simulink library "pixhawk_slib_rfly"  (R2022b)
settings: Solver=ode45  StartTime=0.0  StopTime=10.0  RelTol=1e-3
libraries: pixhawk_slib_uORB_RW x42, $bdroot x7
(part 3 of 3)

== matlab function pixhawk_slib_rfly/PosVelAttAll/quat2eul ==
  data: q input; phi output; theta output; psi output
function [phi,theta,psi] = quat2eul(q)
% Conversion from Quaternion to Euler angles based on the PX4 Firmware
% v1.6.5 release.
% 
% Quaternion -> DCM -> Euler Angles
% INPUT:
%   q: Quaternion vector of the format: (a + bi + cj + dk)
% OUTPUT:
%   [phi,theta,psi]: Euler angles in radians.
% 
 
    a = q(1);
    b = q(2);
    c = q(3);
    d = q(4);

    aSq = a*a;
    bSq = b*b;
    cSq = c*c;
    dSq = d*d;

    d_pi2 = pi/2;

    % quaternion_to_dcm
    dcm00 = aSq + bSq - cSq - dSq;
    % dcm01 = 2*(b*c - a*d);
    dcm02 = 2*(a*c + b*d);
    dcm10 = 2*(b*c + a*d);
    % dcm11 = aSq - bSq + cSq - dSq;
    dcm12 = 2*(c*d - a*b);
    dcm20 = 2*(b*d - a*c);
    dcm21 = 2*(a*b + c*d);
    dcm22 = aSq - bSq - cSq + dSq;

    % dcm_to_euler
    theta = asin(-dcm20);
    if abs(theta - d_pi2) < 1.0e-3
        phi = single(0.0);
        psi = atan2(dcm12, dcm02);
    elseif abs(theta + d_pi2) < 1.0e-3
        phi = single(0.0);
        psi = atan2(-dcm12, -dcm02);
    else
        phi = atan2(dcm21, dcm22);
        psi = atan2(dcm10, dcm00);
    end

end

== matlab function pixhawk_slib_rfly/TorqueThrustCtrls/ArmTrig1 ==
  data: isEn input; cmd output; param1 output; param2 output; param3 output; isSendCmd output; isAutoArm input; isAutoLoiter input; blockMode output
function [cmd,param1,param2,param3,isSendCmd,blockMode] = fcn(isEn,isAutoArm,isAutoLoiter)

persistent lastEnState;
if isempty(lastEnState)
    lastEnState=false;
end


cmd=uint32(0); % 默认空指令
param1=single(0);
param2=single(0);
param3=single(0);
isSendCmd=0; % 不发送

if isEn % 使能的话，就要屏蔽输出
    blockMode=uint8(2); % 如果置于2，则屏蔽力和力矩
else
    blockMode=uint8(0); % 默认不屏蔽输出
end

if isEn~=lastEnState % 不相等，就会触发本循环
    lastEnState=isEn;
    
    if isEn && isAutoArm % 如果开启自动解锁，就解锁飞控
        isSendCmd=1; % 本轮发送
        cmd=uint32(400); %MAV_CMD_COMPONENT_ARM_DISARM，解锁或上锁指令
        param1=single(1); %  Arm 解锁
        param2=single(0); %  No Force 不强制
    end
    
    if ~isEn && isAutoLoiter % 如果开启自动解锁，就解锁飞控
        isSendCmd=1; % 本轮发送
        cmd=uint32(176); %MAV_CMD_DO_SET_MODE 模式设置指令
        param1=single(1); % Mode 设为1，表示确认设置
        param2=single(4); % Custom Mode: PX4_CUSTOM_MAIN_MODE_AUTO 自动模式
        param3=single(3); % Custom Submode: PX4_CUSTOM_SUB_MODE_AUTO_LOITER 悬停子模式
        % 切换到定点模式
        
    end

    
end

== matlab function pixhawk_slib_rfly/OffboardPvaCtrlAPI/CmdGenerator ==
  data: isEnCtrl input; cmd output; params1 output; params2 output; params3 output; isSendCmd output; t input; isSendOff output; isAutoArm input; isAutoBlock input; isSendBlock output; isAutoLoiter input
function [cmd,params1,params2,params3,isSendCmd,isSendOff,isSendBlock] = fcn(isEnCtrl,t,isAutoArm,isAutoBlock,isAutoLoiter)


persistent lastT;
persistent flag;
persistent lastEnCtrl;

isSendBlock=false;

if isempty(lastT)
    lastT=0;
end

if isempty(flag)
    flag=0;
end



if isempty(lastEnCtrl)
    lastEnCtrl=false;
    if isAutoBlock
        isSendBlock=true;
    end
end

isSendCmd=0;
isSendOff=0;

cmd=uint32(0);
params1=single(NaN);
params2=single(NaN);
params3=single(NaN);



if lastEnCtrl~= isEnCtrl% 不相等
    lastEnCtrl = isEnCtrl;
    
    if isAutoBlock
        isSendBlock=true;
    end
    
    
    if isEnCtrl % 使能Offboard
        if isAutoArm
            flag=1; % 进入等待Offboard模式切换指令            
        else
            flag=3; % 直接进入发送数据模式
        end

        
    else % 禁用Offboard
        
        flag=0;
        if isAutoLoiter % 如果启用自动悬停，就进入悬停模式
            isSendCmd=1; % 发送命令
            cmd=uint32(176); %MAV_CMD_DO_SET_MODE
            params1=single(1); % Mode
            params2=single(4); % Custom Mode: PX4_CUSTOM_MAIN_MODE_AUTO
            params3=single(3); % Custom Submode: PX4_CUSTOM_SUB_MODE_AUTO_LOITER
            % 切换到定点模式
        end

    end
    
    lastT=t;
end

if abs(flag-1)<0.01 && (t-lastT)>1.2  % 发送offboard数据2秒后，切换Offboard模式
    flag=2;
    isSendCmd=1; % 发送命令
    cmd=uint32(176); %MAV_CMD_DO_SET_MODE
    params1=single(1); % Mode
    params2=single(6); % Custom Mode: PX4_CUSTOM_MAIN_MODE_OFFBOARD
end


if abs(flag-2)<0.01 && (t-lastT)>2.2  % 切换Offboard1秒后，尝试发送解锁指令
    flag=3;
    isSendCmd=1; % 发送命令
    cmd=uint32(400); %MAV_CMD_COMPONENT_ARM_DISARM
    params1=single(1); %  Arm
    params2=single(0); %  No Force
end

% 只要在Offboard发送模式，就发送Offboard消息
if flag>0.5 && flag<3.5
    isSendOff=1; % 开始发送Offboard消息
end

== matlab function pixhawk_slib_rfly/OffboardAdvCtrlAPI/CmdGenerator ==
  data: isEnCtrl input; cmd output; params1 output; params2 output; params3 output; isSendCmd output; t input; isSendOff output; isAutoArm input; isAutoBlock input; isSendBlock output; isAutoLoiter input
function [cmd,params1,params2,params3,isSendCmd,isSendOff,isSendBlock] = fcn(isEnCtrl,t,isAutoArm,isAutoBlock,isAutoLoiter)


persistent lastT;
persistent flag;
persistent lastEnCtrl;

isSendBlock=false;

if isempty(lastT)
    lastT=0;
end

if isempty(flag)
    flag=0;
end



if isempty(lastEnCtrl)
    lastEnCtrl=false;
    if isAutoBlock
        isSendBlock=true;
    end
end

isSendCmd=0;
isSendOff=0;

cmd=uint32(0);
params1=single(NaN);
params2=single(NaN);
params3=single(NaN);



if lastEnCtrl~= isEnCtrl% 不相等
    lastEnCtrl = isEnCtrl;
    
    if isAutoBlock
        isSendBlock=true;
    end
    
    
    if isEnCtrl % 使能Offboard
        if isAutoArm
            flag=1; % 进入等待Offboard模式切换指令            
        else
            flag=3; % 直接进入发送数据模式
        end

        
    else % 禁用Offboard
        
        flag=0;
        if isAutoLoiter % 如果启用自动悬停，就进入悬停模式
            isSendCmd=1; % 发送命令
            cmd=uint32(176); %MAV_CMD_DO_SET_MODE
            params1=single(1); % Mode
            params2=single(4); % Custom Mode: PX4_CUSTOM_MAIN_MODE_AUTO
            params3=single(3); % Custom Submode: PX4_CUSTOM_SUB_MODE_AUTO_LOITER
            % 切换到定点模式
        end

    end
    
    lastT=t;
end

if abs(flag-1)<0.01 && (t-lastT)>1.2  % 发送offboard数据2秒后，切换Offboard模式
    flag=2;
    isSendCmd=1; % 发送命令
    cmd=uint32(176); %MAV_CMD_DO_SET_MODE
    params1=single(1); % Mode
    params2=single(6); % Custom Mode: PX4_CUSTOM_MAIN_MODE_OFFBOARD
end


if abs(flag-2)<0.01 && (t-lastT)>2.2  % 切换Offboard1秒后，尝试发送解锁指令
    flag=3;
    isSendCmd=1; % 发送命令
    cmd=uint32(400); %MAV_CMD_COMPONENT_ARM_DISARM
    params1=single(1); %  Arm
    params2=single(0); %  No Force
end

% 只要在Offboard发送模式，就发送Offboard消息
if flag>0.5 && flag<3.5
    isSendOff=1; % 开始发送Offboard消息
end

== matlab function pixhawk_slib_rfly/OffboardAdvCtrlAPI/MATLAB Function ==
  data: u input; idxList input; y output
function y = fcn(u,idxList)
y=single(NaN(11,1));
uLen=length(u);
idxLen=length(idxList);

minLen=uLen;
if idxLen<uLen
    minLen=idxLen;
end

if minLen>0.5
    for i=1:minLen
        y(idxList(i))=u(i);
    end
end

== matlab function pixhawk_slib_rfly/OffboardAttCtrlAPI/CmdGenerator ==
  data: isEnCtrl input; cmd output; params1 output; params2 output; params3 output; isSendCmd output; t input; isSendOff output; isAutoArm input; isAutoBlock input; isSendBlock output; isAutoLoiter input
function [cmd,params1,params2,params3,isSendCmd,isSendOff,isSendBlock] = fcn(isEnCtrl,t,isAutoArm,isAutoBlock,isAutoLoiter)


persistent lastT;
persistent flag;
persistent lastEnCtrl;


isSendBlock=false;

if isempty(lastT)
    lastT=0;
end

if isempty(flag)
    flag=0;
end


if isempty(lastEnCtrl)
    lastEnCtrl=false;
    if isAutoBlock
        isSendBlock=true;
    end
end

isSendCmd=0;
isSendOff=0;

cmd=uint16(0);
params1=single(NaN);
params2=single(NaN);
params3=single(NaN);



if lastEnCtrl~= isEnCtrl% 不相等
    lastEnCtrl = isEnCtrl;
    
    if isAutoBlock
        isSendBlock=true;
    end
    
    
    if isEnCtrl % 使能Offboard
        if isAutoArm
            flag=1; % 进入等待Offboard模式切换指令            
        else
            flag=3; % 直接进入发送数据模式
        end
        
    else % 禁用Offboard
        
        flag=0;
        if isAutoLoiter % 如果启用自动悬停，就进入悬停模式
            isSendCmd=1; % 发送命令
            cmd=uint16(176); %MAV_CMD_DO_SET_MODE
            params1=single(1); % Mode
            params2=single(4); % Custom Mode: PX4_CUSTOM_MAIN_MODE_AUTO
            params3=single(3); % Custom Submode: PX4_CUSTOM_SUB_MODE_AUTO_LOITER
            % 切换到定点模式
        end

    end
    
    lastT=t;
end

if abs(flag-1)<0.01 && (t-lastT)>1.2  % 发送offboard数据2秒后，切换Offboard模式
    flag=2;
    isSendCmd=1; % 发送命令
    cmd=uint16(176); %MAV_CMD_DO_SET_MODE
    params1=single(1); % Mode
    params2=single(6); % Custom Mode: PX4_CUSTOM_MAIN_MODE_OFFBOARD
end


if abs(flag-2)<0.01 && (t-lastT)>2.2  % 切换Offboard1秒后，尝试发送解锁指令
    flag=3;
    isSendCmd=1; % 发送命令
    cmd=uint16(400); %MAV_CMD_COMPONENT_ARM_DISARM
    params1=single(1); %  Arm
    params2=single(0); %  No Force
end

% 只要在Offboard发送模式，就发送Offboard消息
if flag>0.5 && flag<3.5
    isSendOff=1; % 开始发送Offboard消息
end
